simulink model "freqspec"  (R2012b)
settings: Solver=ode45  StartTime=0.0  StopTime=1  MaxStep=0.1  RelTol=1e-3
undefined symbols (not defined in the file or in its folder): get, One, sided
libraries: dspsnks4 x2, dspxfrm3 x1, dspsrcs4 x1
settings Model: Creator=Kushal  LastModifiedBy=Kushal

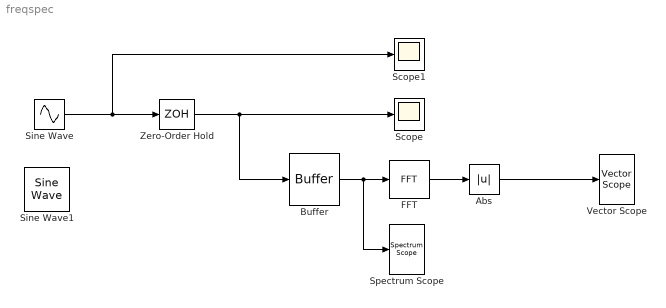
== system freqspec ==
  Abs : Abs
  Buffer : Buffer  N=1024  TreatMby1Signals=One channel
  FFT : dspxfrm3/FFT  CompMethod=Table lookup  TableOpt=NEW  TableOptActive=Speed  BitRevOrder=off  InheritFFTLength=on  FFTLength=64  RowConvenienceOn=on  FFTImplementation=Auto  SkipNorm=off  firstCoeffDataTypeStr=Inherit: Same word length as input  firstCoeffLastDataTypeStr=Inherit: Same word length as input  outputMin=[]  outputMax=[]  roundingMode=Floor  overflowMode=off
  Scope : Scope
      settings: YMin=-1  YMax=1
  Scope1 : Scope
      settings: YMin=-1  YMax=1
  Sine Wave : Sin  Amplitude=1000  Frequency=2*pi*5e3  SampleTime=0
  Sine Wave1 : dspsrcs4/Sine Wave  Amplitude=1  Frequency=100  Phase=0  SampleMode=Discrete  OutComplex=Real  CompMethod=Trigonometric fcn  TableSize=Speed  SampleTime=1/1000  SamplesPerFrame=1  ResetState=Restart at time zero  dataType=double  wordLen=16  udDataType=sfix(16)  fracBitsMode=Best precision  numFracBits=15  OutDataTypeStr=double  LastOutDataTypeStr=double
  Spectrum Scope : dspsnks4/Spectrum Scope  ScopeProperties=on  Domain=Frequency  HorizSpan=1  UseBuffer=off  BufferSize=128  Overlap=0  TreatMby1Signals=One channel  inpFftLenInherit=off  FFTlength=128  numAvg=2  DisplayProperties=off  AxisGrid=on  Memory=off  FrameNumber=on  AxisLegend=off  AxisZoom=off  OpenScopeAtSimStart=on  OpenScopeImmediately=off  FigPos=get(0,'defaultfigureposition')  AxisProperties=off  XUnits=Hertz  XRange=One-sided ([0...Fs/2])  XDisplay=0  InheritXIncr=on  XIncr=1.0  XLabel=Samples  XLimit=Auto  YUnits=dBW/Hertz  XMax=1  XMin=0  YLabel=Magnitude-squared, dB  LineProperties=off  wintypeSpecScope=Hann  RsSpecScope=50  betaSpecScope=5  winsampSpecScope=Periodic  XAxisParamsVer=6.9  isFrameUpgraded=on
      settings: YMin=-10  YMax=10
  Vector Scope : dspsnks4/Vector Scope  ScopeProperties=on  Domain=Frequency  HorizSpan=1  DisplayProperties=off  AxisGrid=on  Memory=off  FrameNumber=on  AxisLegend=off  AxisZoom=off  OpenScopeAtSimStart=on  OpenScopeImmediately=off  FigPos=get(0,'defaultfigureposition')  AxisProperties=off  XUnits=Hertz  XRange=[0...Fs/2]  InheritXIncr=on  XIncr=1  XLabel=Time  XLimit=User-defined  XMin=0  XMax=10000  XStart=0  YUnits=Magnitude  YLabel=Amplitude  LineProperties=off  XAxisParamsVer=6.9
      settings: YMin=-11901.4979  YMax=491871.4476
  Zero-Order Hold : ZeroOrderHold  SampleTime=1e-5
  wires:
  Zero-Order Hold/1 -> Scope/1, Buffer/1
  Buffer/1 -> Spectrum Scope/1, FFT/1
  FFT/1 -> Abs/1
  Abs/1 -> Vector Scope/1
  Sine Wave/1 -> Scope1/1, Zero-Order Hold/1
